simulink model "Automated_solar_tracker"  (R2026a)
settings: Solver=VariableStepAuto  StopTime=20

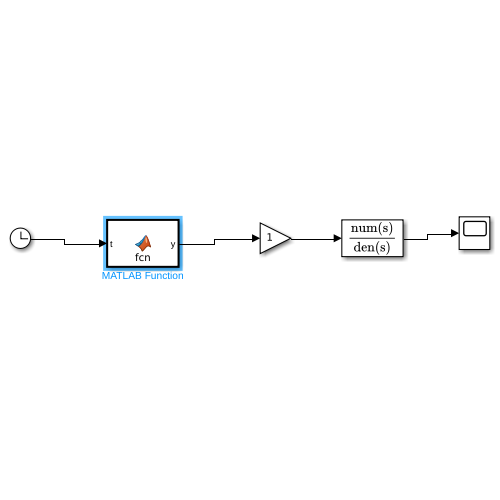
[thumbnail: Simulink's stored preview of the top-level diagram]
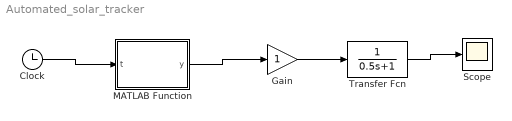
== system Automated_solar_tracker ==
  Clock : Clock
  Gain : Gain
  MATLAB Function : MATLAB Function  TreatAsAtomicUnit=on
  Scope : Scope
  Transfer Fcn : TransferFcn  Denominator=[0.5 1]
  wires:
  Clock/1 -> MATLAB Function/1(t)
  MATLAB Function/1(y) -> Gain/1
  Gain/1 -> Transfer Fcn/1
  Transfer Fcn/1 -> Scope/1

== matlab function Automated_solar_tracker/MATLAB Function ==
  data: t input; y output
function y = fcn(t)

if t < 6
    y = 0;
elseif t > 18
    y = 180;
else
    y = (t - 6) * 15;
end

end
